simulink model "E2_Simulink"  (R2022b)
settings: Solver=VariableStepAuto  StartTime=0.0  StopTime=10.0  MaxStep=0.0001  RelTol=1e-3
values from neighbouring files (symbols this model uses):
  k = 100    [E2_Parametros.m]
  m = 10    [E2_Parametros.m]
  r = 0.05    [E2_Parametros.m]
settings Model: Creator=mluser  LastModifiedBy=mluser

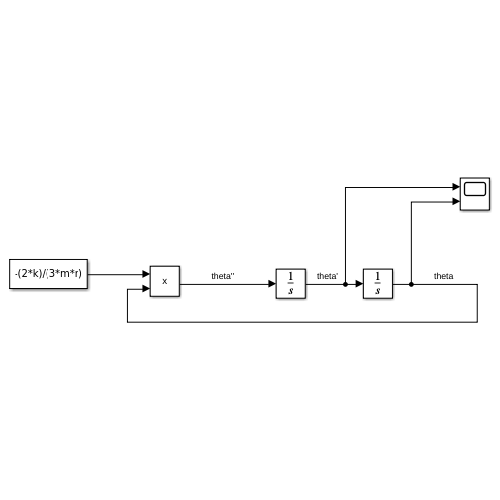
[thumbnail: Simulink's stored preview of the top-level diagram]
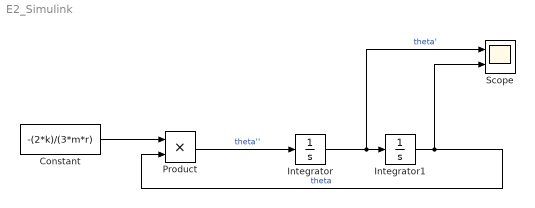
== system E2_Simulink ==
  Constant : Constant  Value=-(2*k)/(3*m*r)
  Integrator : Integrator
  Integrator1 : Integrator  InitialCondition=20*(pi/180)
  Product : Product
  Scope : Scope  NumInputPorts=2
  wires:
  Integrator/1 -> Scope/1, Integrator1/1  "theta'"
  Product/1 -> Integrator/1  "theta''"
  Constant/1 -> Product/1
  Integrator1/1 -> Scope/2, Product/2  "theta"
